simulink model "TemperatureControl"  (R2020a)
settings: Solver=VariableStepAuto  StartTime=0.0  StopTime=10.0  RelTol=1e-3
settings Model: Creator=julius  LastModifiedBy=julius

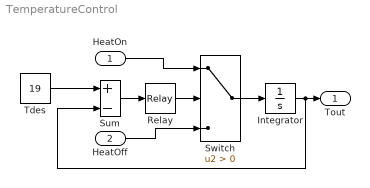
== system TemperatureControl ==
  HeatOn : Inport
  HeatOff : Inport  Port=2
  Integrator : Integrator
  Relay : Relay  OnSwitchValue=0.5  OffSwitchValue=-0.5
  Sum : Sum  Inputs=+-
  Switch : Switch  Criteria=u2 > Threshold
  Tdes : Constant  Value=19
  Tout : Outport
  wires:
  Tdes/1 -> Sum/1
  Sum/1 -> Relay/1
  Relay/1 -> Switch/2
  HeatOn/1 -> Switch/1
  HeatOff/1 -> Switch/3
  Switch/1 -> Integrator/1
  Integrator/1 -> Sum/2, Tout/1
